simulink model "exercise00_superposition"  (R2022a)
settings: Solver=VariableStepAuto  StartTime=0.0  StopTime=30  RelTol=1e-3
settings Model: Creator=ac133867  LastModifiedBy=cunis
settings DebuggingCC: UnconnectedInputMsg=warning  UnconnectedOutputMsg=warning  UnconnectedLineMsg=warning
settings RTWCC: DLArmComputeVersion=19.05

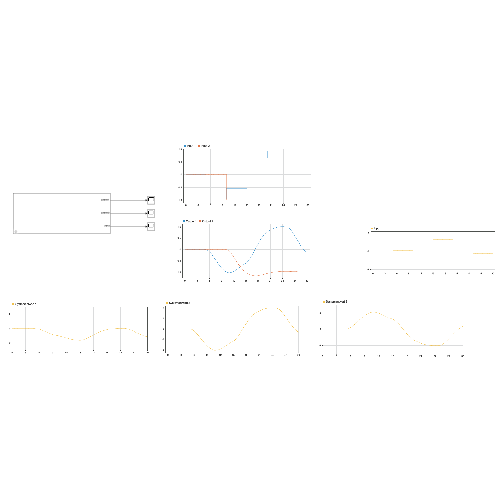
[thumbnail: Simulink's stored preview of the top-level diagram]
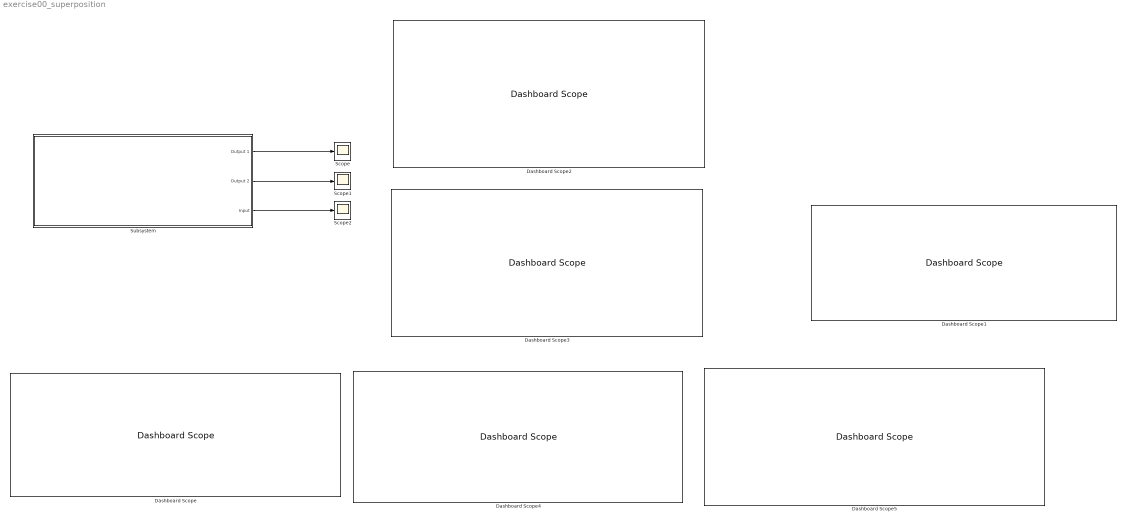
== system exercise00_superposition ==
  Dashboard Scope{,1..5} (6 alike) : DashboardScope
  Scope : Scope
  Scope1 : Scope
  Scope2 : Scope
  Subsystem : Subsystem
      mask DialogControl Control2 Prompt: Simulate Subsystems
  wires:
  Subsystem/1(Output 1) -> Scope/1
  Subsystem/2(Output 2) -> Scope1/1
  Subsystem/3(Input) -> Scope2/1

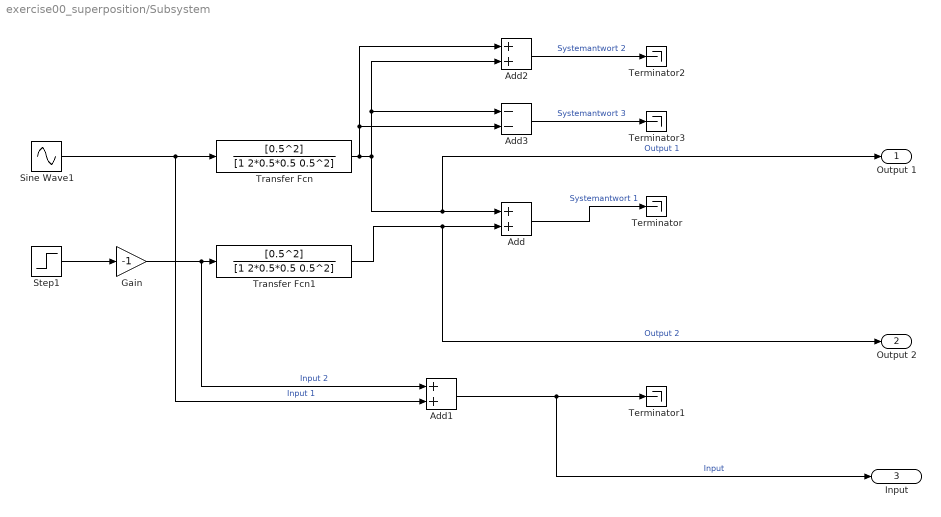
== system exercise00_superposition/Subsystem ==
  Add : Sum
  Add1 : Sum
  Add2 : Sum
  Add3 : Sum  Inputs=--
  Gain : Gain  Gain=-1
  Sine Wave1 : Sin  SampleTime=5
  Step1 : Step  Time=10  SampleTime=0
  Terminator{,1..3} (4 alike) : Terminator
  Transfer Fcn : TransferFcn  Numerator=[0.5^2]  Denominator=[1 2*0.5*0.5 0.5^2]
  Transfer Fcn1 : TransferFcn  Numerator=[0.5^2]  Denominator=[1 2*0.5*0.5 0.5^2]
  Output 1 : Outport
  Output 2 : Outport  Port=2
  Input : Outport  Port=3
  wires:
  Sine Wave1/1 -> Transfer Fcn/1, Add1/2  "Input 1"
  Transfer Fcn/1 -> Add3/2, Add2/1, Add3/1, Add2/2, Output 1/1, Add/1  "Output 1"
  Add1/1 -> Input/1, Terminator1/1  "Input"
  Transfer Fcn1/1 -> Output 2/1, Add/2  "Output 2"
  Gain/1 -> Add1/1, Transfer Fcn1/1  "Input 2"
  Step1/1 -> Gain/1
  Add/1 -> Terminator/1  "Systemantwort 1"
  Add2/1 -> Terminator2/1  "Systemantwort 2"
  Add3/1 -> Terminator3/1  "Systemantwort 3"
